simulink model "rtwdemo_tflmath"  (Simulink 7.6)
settings: Solver=FixedStepDiscrete  StartTime=0.0  StopTime=1  FixedStep=1  RelTol=1e-3  SampleTimeConstraint=Specified
PreLoadFcn:
  | addpath(fullfile(matlabroot,'toolbox','rtw','rtwdemos','tfl_demo'));
  | sl_refresh_customizations;
libraries: rtwdemowidgets x2
settings Model: Creator=The MathWorks Inc.  ExtModeAutoUpdateStatusClock=off
settings MATStruct: SampleTime=1  Offset=0  Priority=[30.0]
settings DataIOCC: SaveFormat=StructureWithTime  SaveOutput=off  SaveTime=off
settings OptimizationCC: InlineParams=on  InlineInvariantSignals=on  MemcpyThreshold=5  PassReuseOutputArgsAs=Individual arguments  StateBitsets=on  DataBitsets=on  UseTempVars=on  ZeroExternalMemoryAtStartup=off  ZeroInternalMemoryAtStartup=off  NoFixptDivByZeroProtection=on  EfficientFloat2IntCast=on  EfficientMapNaN2IntZero=off  OptimizeModelRefInitCode=on  LifeSpan=1
settings DebuggingCC: StrictBusMsg=ErrorOnBusTreatedAsVector
settings HardwareCC: ProdBitPerLong=64  ProdEndianess=LittleEndian  ProdWordSize=64  ProdHWDeviceType=Specified  TargetHWDeviceType=32-bit Generic
settings SFSimCC: SimParseCustomCode=off
settings RTWCC: SystemTargetFile=ert.tlc  GenCodeOnly=on  TemplateMakefile=ert_default_tmf  Description=Real-Time Workshop Embedded Coder (no auto configuration)  GenerateReport=on  RTWVerbose=off  ProcessScript=ert_make_rtw_hook  IncludeHyperlinkInReport=on  LaunchReport=on  GenerateTraceInfo=on  GenerateTraceReport=on  GenerateTraceReportSl=on  GenerateTraceReportSf=on  GenerateTraceReportEml=on
settings CodeAppCC: ForceParamTrailComments=on  IgnoreCustomStorageClasses=off  IgnoreTestpoints=on  SimulinkDataObjDesc=on  CustomSymbolStrGlobalVar=rt$N$M  CustomSymbolStrType=$N$M  CustomSymbolStrFcn=$N$M$F  CustomSymbolStrMacro=$N$M  InsertBlockDesc=on
settings ERTTargetCC: TargetFunctionLibrary=Math Function Examples  MultiwordLength=2048  GenerateSampleERTMain=on  IncludeMdlTerminateFcn=off  SupportComplex=off  InlinedParameterPlacement=NonHierarchical  ERTCustomFileTemplate=example_file_process.tlc  ConvertIfToSwitch=off

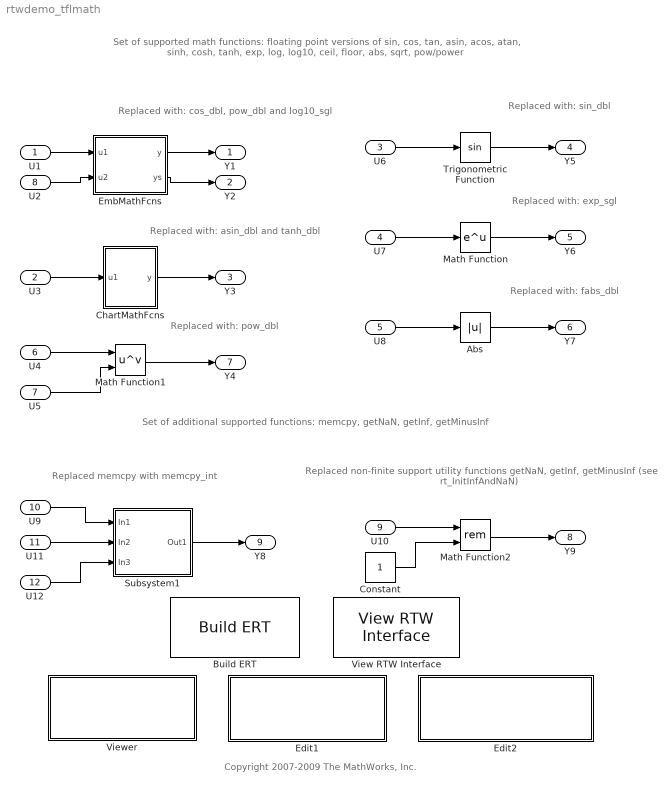
== system rtwdemo_tflmath ==
  note: Copyright 2007-2009 The MathWorks, Inc.
  note: Set of supported math functions:
      | floating point versions of
      | sin, cos, tan, asin, acos, atan, sinh, cosh, tanh,
      | exp, log, log10, ceil, floor, abs, sqrt, pow/power
  note: Replaced with:
      | cos_dbl, pow_dbl and log10_sgl
  note: Replaced with:
      | asin_dbl and tanh_dbl
  note: Replaced with:
      | sin_dbl
  note: Replaced with:
      | exp_sgl
  note: Replaced with:
      | fabs_dbl
  note: Replaced with:
      | pow_dbl
  note: Replaced non-finite support utility functions
      | getNaN, getInf, getMinusInf
      | (see rt_InitInfAndNaN)
  note: Replaced memcpy with memcpy_int
  note: Set of additional supported functions:
      | memcpy, getNaN, getInf, getMinusInf
  U1 : Inport  OutDataTypeStr=double  PortDimensions=1  SampleTime=1
  U3 : Inport  Port=2
  U6 : Inport  Port=3  OutDataTypeStr=double  PortDimensions=1  SampleTime=1
  U7 : Inport  Port=4  OutDataTypeStr=single  PortDimensions=1  SampleTime=1
  U8 : Inport  Port=5  OutDataTypeStr=double  PortDimensions=1  SampleTime=1
  U4 : Inport  Port=6  OutDataTypeStr=double  PortDimensions=1  SampleTime=1
  U5 : Inport  Port=7  OutDataTypeStr=double  PortDimensions=1  SampleTime=1
  U2 : Inport  Port=8  OutDataTypeStr=double  PortDimensions=1  SampleTime=1
  U10 : Inport  Port=9  OutDataTypeStr=double  PortDimensions=1  SampleTime=1
  U9 : Inport  Port=10  OutDataTypeStr=int32  PortDimensions=[1,100]  SampleTime=1
  U11 : Inport  Port=11  OutDataTypeStr=int32  PortDimensions=[1,100]  SampleTime=1
  U12 : Inport  Port=12  OutDataTypeStr=int32  PortDimensions=[1,100]  SampleTime=1
  Abs : Abs
  Build ERT : rtwdemowidgets/Build ERT  SystemSampleTime=-1  attrib_overrides={'GenFloatMathFcnCalls','SupportNonFinite'}
  ChartMathFcns : Stateflow chart  TreatAsAtomicUnit=on
  Constant : Constant  OutDataTypeStr=double
  Edit1 : Subsystem  mask{attrib_overrides={}}
      mask prompts: attrib_overrides "List of attributes to preserve (cell of strings):"
      mask help: Enter the attributes of the configuration set that you want preserved. Otherwise, the default configuration script will override your current settings.
      settings: OpenFcn=edit('tfl_table_math');
      mask Display:
      | disp(['View/edit TFL Definition\n',...
      | 	  'tfl_table_math.m\n(double-click)'])
  Edit2 : Subsystem  mask{attrib_overrides={}}
      mask prompts: attrib_overrides "List of attributes to preserve (cell of strings):"
      mask help: Enter the attributes of the configuration set that you want preserved. Otherwise, the default configuration script will override your current settings.
      settings: OpenFcn=edit(fullfile(matlabroot,'toolbox','rtw','rtwdemos','tfl_demo', 'sl_customization.m'));
      mask Display:
      | disp(['View/edit TFL Registration\n',...
      | 	  'sl_customization.m\n(double-click)'])
  EmbMathFcns : Stateflow chart  TreatAsAtomicUnit=on
  Math Function : Math  SaturateOnIntegerOverflow=on
  Math Function1 : Math  Operator=pow  SaturateOnIntegerOverflow=on
  Math Function2 : Math  Operator=rem  SaturateOnIntegerOverflow=on
  Subsystem1 : Subsystem  TreatAsAtomicUnit=on
  Trigonometric Function : Trigonometry
  View RTW Interface : rtwdemowidgets/View RTW Interface  SystemSampleTime=-1
  Viewer : Subsystem  mask{attrib_overrides={}}
      mask prompts: attrib_overrides "List of attributes to preserve (cell of strings):"
      mask help: Enter the attributes of the configuration set that you want preserved. Otherwise, the default configuration script will override your current settings.
      settings: OpenFcn=|
      | tfl = tfl_table_math;
      | obj = RTW.viewTfl(tfl);
      | clear tfl obj;
      mask Display:
      | disp(['Invoke TFL Viewer on\n',...
      | 	  'tfl_table_math.m\n(double-click)'])
  Y1 : Outport
  Y2 : Outport  Port=2
  Y3 : Outport  Port=3
  Y5 : Outport  Port=4
  Y6 : Outport  Port=5
  Y7 : Outport  Port=6
  Y4 : Outport  Port=7
  Y9 : Outport  Port=8
  Y8 : Outport  Port=9
  wires:
  U1/1 -> EmbMathFcns/1(u1)
  EmbMathFcns/1(y) -> Y1/1
  EmbMathFcns/2(ys) -> Y2/1
  U3/1 -> ChartMathFcns/1(u1)
  ChartMathFcns/1(y) -> Y3/1
  U6/1 -> Trigonometric Function/1
  Trigonometric Function/1 -> Y5/1
  U7/1 -> Math Function/1
  Math Function/1 -> Y6/1
  U8/1 -> Abs/1
  Abs/1 -> Y7/1
  U4/1 -> Math Function1/1
  Math Function1/1 -> Y4/1
  U5/1 -> Math Function1/2
  U2/1 -> EmbMathFcns/2(u2)
  U10/1 -> Math Function2/1
  Math Function2/1 -> Y9/1
  Constant/1 -> Math Function2/2
  Subsystem1/1(Out1) -> Y8/1
  U9/1 -> Subsystem1/1(In1)
  U11/1 -> Subsystem1/2(In2)
  U12/1 -> Subsystem1/3(In3)

== system rtwdemo_tflmath/Edit1 ==

== system rtwdemo_tflmath/Edit2 ==

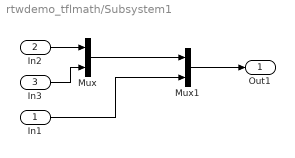
== system rtwdemo_tflmath/Subsystem1 ==
  In1 : Inport
  In2 : Inport  Port=2
  In3 : Inport  Port=3
  Mux : Mux  Inputs=2
  Mux1 : Mux  Inputs=2
  Out1 : Outport
  wires:
  In1/1 -> Mux1/2
  In3/1 -> Mux/2
  In2/1 -> Mux/1
  Mux1/1 -> Out1/1
  Mux/1 -> Mux1/1

== system rtwdemo_tflmath/Viewer ==

== stateflow chart ChartMathFcns ==
  (default) -> (junction 3) : {y := asin(u1) +tanh(u1);}
  data: u1 input uint16; y output uint16

== matlab function EmbMathFcns ==
  data: u1 input double; y output double; ys output double; u2 input double
function [y,ys] = fcn(u1,u2)
% This block supports the Embedded MATLAB subset.
% See the help menu for details. 

    u1s = single(u1);
    
    y = cos(u1) + power(u1, u2);
    ys = log10(u1s);
end
